simulink model "Final_System"  (R2025b)
settings: Solver=FixedStepDiscrete  StartTime=0.0  StopTime=20.0  FixedStep=0.01  RelTol=1e-3
undefined symbols (not defined in the file): DiscIntNeverNeededParam
libraries: simulink x2, slpidlib x1
settings Model: Creator=ramal  LastModifiedBy=kiaza
settings HardwareCC: TargetBitPerPointer=64.0  TargetBitPerSizeT=64.0  TargetBitPerPtrDiffT=64.0  TargetLongLongMode=on  TargetIntDivRoundTo=Zero  TargetEndianess=LittleEndian  TargetWordSize=64.0  TargetHWDeviceType=MATLAB Host  ProdEqTarget=off
settings RTWCC: GenCodeOnly=on  TemplateMakefile=RTW.MSVCBuild  GenerateReport=on  LaunchReport=on  Description=Create Visual C/C++ Solution File for Simulink Coder

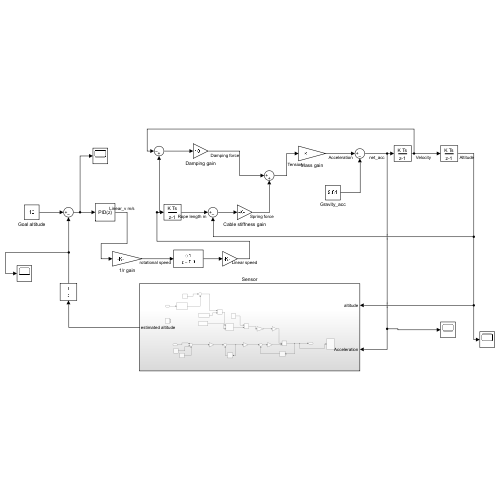
[thumbnail: Simulink's stored preview of the top-level diagram]
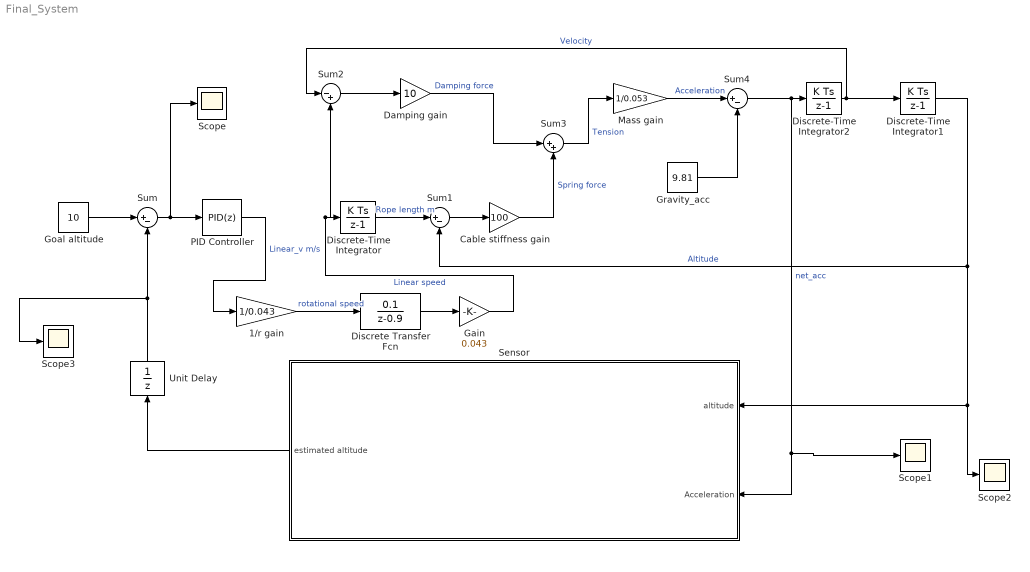
== system Final_System ==
  1/r gain : Gain  Gain=1/0.043
  Cable stiffness gain : Gain  Gain=100
  Damping gain : Gain  Gain=10
  Discrete Transfer Fcn : DiscreteTransferFcn  Numerator=[0.1]  Denominator=[1 -0.9]
  Discrete-Time Integrator : DiscreteIntegrator  SampleTime=0.01  ICPrevOutput=DiscIntNeverNeededParam  ICPrevScaledInput=DiscIntNeverNeededParam
  Discrete-Time Integrator1 : DiscreteIntegrator  SampleTime=0.01  ICPrevOutput=DiscIntNeverNeededParam  ICPrevScaledInput=DiscIntNeverNeededParam
  Discrete-Time Integrator2 : DiscreteIntegrator  SampleTime=0.01  ICPrevOutput=DiscIntNeverNeededParam  ICPrevScaledInput=DiscIntNeverNeededParam
  Gain : Gain  Gain=0.043
  Goal altitude : Constant  Value=10
  Gravity_acc : Constant  Value=9.81
  Mass gain : Gain  Gain=1/0.053
  PID Controller : slpidlib/PID Controller  Controller=PID  Form=Parallel  TimeDomain=Discrete-time  UseExternalTs=off  SampleTime=-1  IntegratorMethod=Forward Euler  FilterMethod=Forward Euler  ControllerParametersSource=internal  P=1  I=0.2  UseKiTs=off  D=0.1  UseExternalDerivativeSource=off  N=100  UseFilter=on  TunerSelectOption=Transfer Function Based (PID Tuner App)  InitialConditionSource=internal  InitialConditionForIntegrator=0  InitialConditionForFilter=0  DifferentiatorICPrevScaledInput=0  ExternalReset=none  TrackingMode=off  Kt=1  LimitOutput=off  SatLimitsSource=internal  UpperSaturationLimit=inf  LowerSaturationLimit=-inf  LinearizeAsGain=on  AntiWindupMode=none  Kb=1  LimitIntegrator=off  UpperIntegratorSaturationLimit=inf  LowerIntegratorSaturationLimit=-inf  POutMin=[]  POutMax=[]  IOutMin=[]  IOutMax=[]  DOutMin=[]  DOutMax=[]  NOutMin=[]  NOutMax=[]  SumOutMin=[]  SumOutMax=[]  SaturationOutMin=[]  SaturationOutMax=[]  PParamMin=[]  PParamMax=[]  IParamMin=[]  IParamMax=[]  DParamMin=[]  DParamMax=[]  NParamMin=[]  NParamMax=[]  KbParamMin=[]  KbParamMax=[]  KtParamMin=[]  KtParamMax=[]  KbOutMin=[]  KbOutMax=[]  KtOutMin=[]  KtOutMax=[]  IntegratorOutMin=[]  IntegratorOutMax=[]  FilterOutMin=[]  FilterOutMax=[]  SumI1OutMin=[]  SumI1OutMax=[]  SumI2OutMin=[]  SumI2OutMax=[]  SumI3OutMin=[]  SumI3OutMax=[]  SumI4OutMin=[]  SumI4OutMax=[]  SumDOutMin=[]  SumDOutMax=[]  DifferentiatorOutMin=[]  DifferentiatorOutMax=[]  FilterDiffOutCoefMin=[]  FilterDiffOutCoefMax=[]  ReciprocalOutMin=[]  ReciprocalOutMax=[]  SumDenOutMin=[]  SumDenOutMax=[]  SumNumOutMin=[]  SumNumOutMax=[]  DivideOutMin=[]  DivideOutMax=[]  UdiffTsProdOutMin=[]  UdiffTsProdOutMax=[]  NTsProdOutMin=[]  NTsProdOutMax=[]  UintegralTsProdOutMin=[]  UintegralTsProdOutMax=[]  UngainTsProdOutMin=[]  UngainTsProdOutMax=[]  ClampingZeroOutDataTypeStr=Inherit: Inherit via back propagation  ClampingZeroOutMin=[]  ClampingZeroOutMax=[]  FilterDenConstantOutDataTypeStr=Inherit: Inherit via back propagation  FilterDenConstantOutMin=[]  FilterDenConstantOutMax=[]  PCopyOutDataTypeStr=Inherit: Inherit via back propagation  PCopyOutMin=[]  PCopyOutMax=[]  NCopyOutDataTypeStr=Inherit: Inherit via back propagation  NCopyOutMin=[]  NCopyOutMax=[]  IntegratorContinuousStateAttributes=''  IntegratorStateMustResolveToSignalObject=off  IntegratorRTWStateStorageClass=Auto  FilterContinuousStateAttributes=''  FilterStateMustResolveToSignalObject=off  FilterRTWStateStorageClass=Auto  ParallelPVariant=InternalParameters  IdealPVariant=Disabled  IVariant=InternalParameters  DVariant=InternalParameters  IntegratorVariant=Discrete  SatVariant=Disabled  AWVariant=Passthrough  PCopyVariant=Disabled  TRVariant=Disabled  FdbkBlocksVariant=Forward  IdealPFdbkVariant=Disabled  SatFdbkVariant=Disabled  DerivativeFilterVariant=ForwardEulerFilter  NVariant=InternalParameters  NCopyVariant=Disabled  FilterICVariant=InternalICsFilter  IntegratorICVariant=InternalICs  ExternalResetVariant=Disabled  TRSumVariant=Passthrough  SumFdbkVariant=Disabled  SumVariant=Sum_PID  TsampFilterVariant=InternalTs  TsampNgainVariant=Passthrough  TsampIntegralVariant=Disabled_SignalSpec  ExternalSaturationOutDataTypeStr=Inherit: Same as second input  DerivativeSourceVariant=ErrorSignal  PreIntVariant=InternalPreInt
  Scope{,1..3} (4 alike) : Scope
      Scope settings: ActiveDisplayYMinimum=-2.76085  ActiveDisplayYMaximum=11.42823
      Scope1 settings: ActiveDisplayYMinimum=-2122.83033  ActiveDisplayYMaximum=2551.61574  DataLoggingVariableName=ScopeData3
      Scope2 settings: ActiveDisplayYMinimum=-1.38709  ActiveDisplayYMaximum=12.47397  DataLoggingVariableName=ScopeData2
      Scope3 settings: ActiveDisplayYMinimum=-1.42823  ActiveDisplayYMaximum=12.76085  DataLoggingVariableName=ScopeData5
  Sensor : Subsystem
  Sum : Sum  Inputs=|+-
  Sum1 : Sum  Inputs=|+-
  Sum2 : Sum  Inputs=|-+
  Sum3 : Sum  Inputs=|++
  Sum4 : Sum  Inputs=|+-
  Unit Delay : UnitDelay  SampleTime=-1  HasFrameUpgradeWarning=on
  wires:
  Goal altitude/1 -> Sum/1
  Sum/1 -> Scope/1, PID Controller/1
  Discrete-Time Integrator/1 -> Sum1/1  "Rope length m"
  Sum1/1 -> Cable stiffness gain/1
  Sum2/1 -> Damping gain/1
  Cable stiffness gain/1 -> Sum3/2  "Spring force"
  Damping gain/1 -> Sum3/1  "Damping force"
  Sum3/1 -> Mass gain/1  "Tension"
  Discrete-Time Integrator2/1 -> Sum2/1, Discrete-Time Integrator1/1  "Velocity"
  Discrete-Time Integrator1/1 -> Sum1/2, Scope2/1, Sensor/1(altitude)  "Altitude"
  Mass gain/1 -> Sum4/1  "Acceleration"
  Gravity_acc/1 -> Sum4/2
  Sum4/1 -> Discrete-Time Integrator2/1, Scope1/1, Sensor/2(Acceleration)  "net_acc"
  Sensor/1(estimated altitude) -> Unit Delay/1
  Unit Delay/1 -> Scope3/1, Sum/2
  Discrete Transfer Fcn/1 -> Gain/1
  Gain/1 -> Sum2/2, Discrete-Time Integrator/1  "Linear speed"
  1/r gain/1 -> Discrete Transfer Fcn/1  "rotational speed"
  PID Controller/1 -> 1/r gain/1  "Linear_v m/s"

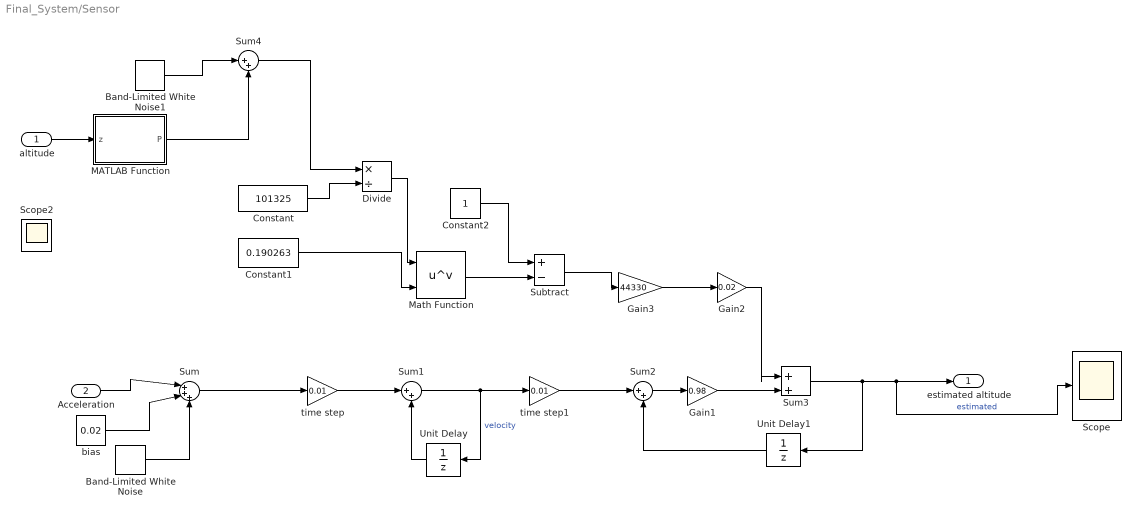
== system Final_System/Sensor ==
  altitude : Inport
  Acceleration : Inport  Port=2
  Band-Limited White Noise : simulink/Sources/Band-Limited White Noise  Cov=[0.01]  Ts=0.01  seed=[23341]
  Band-Limited White Noise1 : simulink/Sources/Band-Limited White Noise  Cov=[2]  Ts=0.01  seed=[23341]
  Constant : Constant  Value=101325
  Constant1 : Constant  Value=0.190263
  Constant2 : Constant
  Divide : Product  Inputs=*/
  Gain1 : Gain  Gain=0.98
  Gain2 : Gain  Gain=0.02
  Gain3 : Gain  Gain=44330
  MATLAB Function : MATLAB Function  TreatAsAtomicUnit=on
  Math Function : Math  Operator=pow
  Scope : Scope
      settings: ActiveDisplayYMinimum=-1.42823  ActiveDisplayYMaximum=12.76085
  Scope2 : Scope  NumInputPorts=2
      settings: ActiveDisplayYMinimum=-1  ActiveDisplayYMaximum=1  DataLoggingVariableName=ScopeData4
  Subtract : Sum  Inputs=+-
  Sum : Sum  Inputs=|+++
  Sum{1..4} (4 alike) : Sum  Inputs=|++
  Unit Delay : UnitDelay  SampleTime=0.01  HasFrameUpgradeWarning=on
  Unit Delay1 : UnitDelay  SampleTime=0.01  HasFrameUpgradeWarning=on
  bias : Constant  Value=0.02
  time step : Gain  Gain=0.01
  time step1 : Gain  Gain=0.01
  estimated altitude : Outport
  wires:
  Math Function/1 -> Subtract/2
  time step/1 -> Sum1/1
  Sum1/1 -> time step1/1, Unit Delay/1  "velocity"
  Constant2/1 -> Subtract/1
  Constant/1 -> Divide/2
  Constant1/1 -> Math Function/2
  Sum3/1 -> Scope/1, estimated altitude/1, Unit Delay1/1  "estimated"
  Unit Delay1/1 -> Sum2/2
  Gain3/1 -> Gain2/1
  Sum2/1 -> Gain1/1
  time step1/1 -> Sum2/1
  Unit Delay/1 -> Sum1/2
  Subtract/1 -> Gain3/1
  Gain2/1 -> Sum3/1
  Divide/1 -> Math Function/1
  Gain1/1 -> Sum3/2
  altitude/1 -> MATLAB Function/1(z)
  bias/1 -> Sum/2
  Band-Limited White Noise/1 -> Sum/3
  Band-Limited White Noise1/1 -> Sum4/1
  MATLAB Function/1(P) -> Sum4/2
  Sum4/1 -> Divide/1
  Acceleration/1 -> Sum/1
  Sum/1 -> time step/1

== matlab function Final_System/Sensor/MATLAB Function ==
  data: z input; P output
function P = alt_to_pres(z)

% Constants (ISA approximation)
P0 = 101325;   % sea level pressure [Pa]
H  = 8400;     % scale height [m]

% Ensure altitude is valid
if z < 0
    z = 0;
end

% Barometric formula
P = P0 * exp(-z / H);

end
